simulink model "StartBlock"  (R2021b)
settings: Solver=VariableStepAuto  StartTime=0.0  StopTime=168  RelTol=1e-3  EnableMultiTasking=on
InitFcn:
  | % Load the model which describes
  | % the traffic flow throughout the
  | % day.
  | %load("TrafficFlowModel.Mat")
  | 
  | % Load the values at each quarter,
  | % Sufficient for traffic modelling.
  | load("TrafficFlowValues.mat")
undefined symbols (not defined in the file or in its folder): m, n, WhichPort
settings Model: Creator=Konrad  LastModifiedBy=Theodor Jonsson
settings SolverCC: AlgebraicLoopSolver=TrustRegion
settings DataIOCC: ReturnWorkspaceOutputs=off
settings OptimizationCC: LifeSpan=inf
settings DebuggingCC: SFUnexpectedBacktrackingDiag=warning  SFNoUnconditionalDefaultTransitionDiag=warning  SFExecutionAtInitializationDiag=none  SFMachineParentedDataDiag=warning  ArithmeticOperatorsInVariantConditions=warning
settings SFSimCC: SimUseLocalCustomCode=off  CustomCodeUndefinedFunction=UseInterfaceOnly
settings RTWCC: RTWUseLocalCustomCode=off
settings CodeAppCC: StateflowObjectComments=on
settings GRTTargetCC: TargetLangStandard=C89/C90 (ANSI)
settings ConfigComp: CovMetricSettings=dw  CovSaveCumulativeToWorkspaceVar=on  CovSaveSingleToWorkspaceVar=on  CovExternalEMLEnable=off

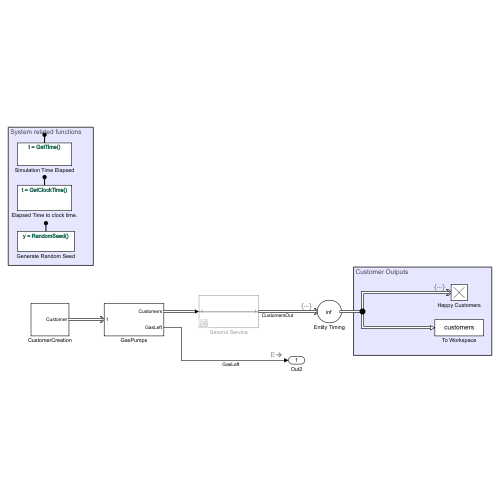
[thumbnail: Simulink's stored preview of the top-level diagram]
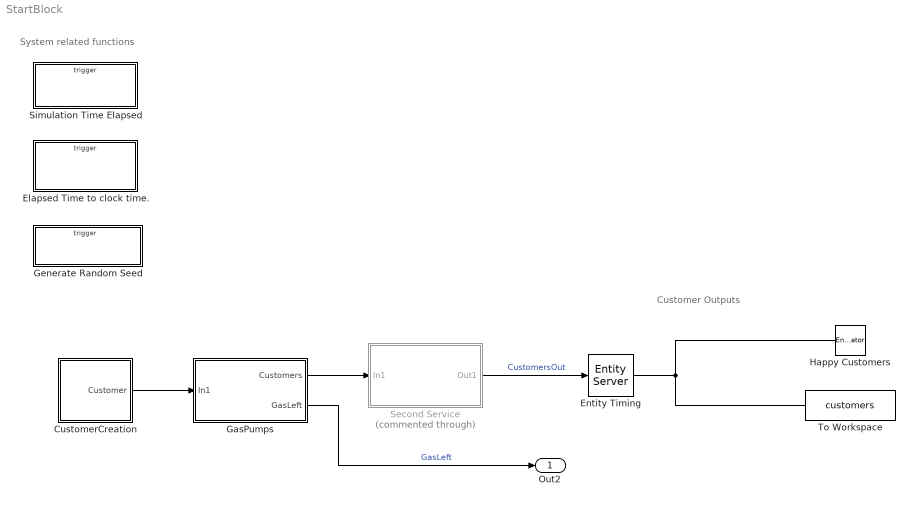
== system StartBlock ==
  note: Customer Outputs
  note: System related functions
  CustomerCreation : Subsystem  mask{mu_passengers=1.45, hunger_prob=0.4, mu_customers=150}
      mask prompts: mu_passengers "Average number of passengers"; hunger_prob "Probability one passenger hungry"; mu_customers "Arriving Customers per hour"
      mask DialogControl DescGroupVar Prompt: Entity Creation
  Elapsed Time to clock time. : Subsystem  TreatAsAtomicUnit=on
  Entity Timing : EntityServer  InputPortMessageModes=m  OutputPortMessageModes=m  Capacity=inf  ServiceTimeValue=0  EntryAction=entity.ServiceTime = GetTime()-entity.ServiceTime;
  GasPumps : Subsystem  mask{n_pumps=20, pump_rate=1200, tank_size=800000, que_cap=2}
      mask prompts: n_pumps "# Pumps"; pump_rate "Pump rate (l/h)"; tank_size "Tank Size"; que_cap "Per pump que capacity"
      mask DialogControl DescGroupVar Prompt: Gas Station
  Generate Random Seed : Subsystem  TreatAsAtomicUnit=on
  Happy Customers : EntityTerminator  InputPortMessageModes=m  EntryAction=entity.ServiceTime = GetTime()-entity.ServiceTime;
  Second Service : Subsystem  Commented=through
  Simulation Time Elapsed : Subsystem  TreatAsAtomicUnit=on
  To Workspace : ToWorkspace  VariableName=customers  SaveFormat=Timeseries  SampleTime=-1
  Out2 : Outport
  wires:
  GasPumps/1(Customers) -> Second Service/1(In1)
  Second Service/1(Out1) -> Entity Timing/1  "CustomersOut"
  GasPumps/2(GasLeft) -> Out2/1  "GasLeft"
  Entity Timing/1 -> Happy Customers/1, To Workspace/1
  CustomerCreation/1(Customer) -> GasPumps/1(In1)

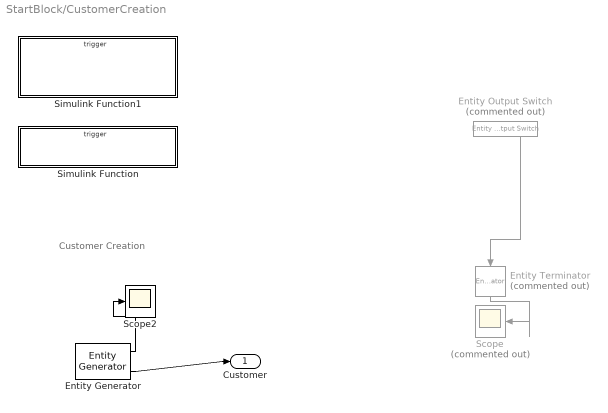
== system StartBlock/CustomerCreation ==
  note: Customer Creation
  Entity Output Switch : EntityOutputSwitch  Commented=on  InputPortMessageModes=m,m  OutputPortMessageModes=m,m  SwitchingCriterion=From control port  SwitchAttributeName=RequiredGas
      settings: InputPortMap=u0,u1
  Entity Generator : EntityGenerator  OutputPortMessageModes=n,m  TimeSource=MATLAB action  Period=1/4  IntergenerationTimeAction=|  GenerateAction=|  AttributeName=Vehicle|Passengers|RequiredGas|Hungry|ServiceTime  AttributeInitialValue=1|1|1|1|0  NumberEntitiesDeparted=on  EntityType=Structured  EntityTypeName=Customer
      IntergenerationTimeAction=|
      | seed = RandomSeed();
      | rng(seed);
      | dt = exprnd(1/(mu_customers*CustomerFrequency()+eps),1);
      GenerateAction=|
      | seed = RandomSeed();
      | rng(seed);
      | vehicle = GenerateVehicle(); % 1 for gas vehicle, 0 for non gas.
      | % In europe the average car occupies 1.5 passengers.
      | % Therefor sample from weighted descrete variable.
      | passengers = max(poissrnd(mu_passengers),1);
      | % Gas required.
      | if vehicle==1 % Car
      |     required_gas = normrnd(45,4);
      | elseif vehicle==2 % Trucks
      |     required_gas = normrnd(757,40);
      | else % Pedestrians don't need gas.
      |     required_gas = 0;
      | end
      | 
      | % Probability of buying snacks increases with the 
      | % amount of passengers and the time of day.
      | % Mid day low, Midnight high probability.
      | 
      | % Assuming that each person has a 25% chance of
      | % wanting buy snacks. Approve snacks attempt if 
      | % more than half of the passengers want to buy snacks.
      | 
      | hungry = binornd(passengers,hunger_prob)>=ceil(passengers/2);
      | % Described in words this checks if more or equal to half
      | % of the passengers are hungry given a probability p of hunger.
      | entity.Vehicle = vehicle;
      | entity.Passengers = passengers;
      | entity.RequiredGas = required_gas;
      | entity.Hungry = double(hungry);
      settings: OutputPortMap=o0,o3
  Entity Terminator : EntityTerminator  Commented=on  InputPortMessageModes=m  NumberEntitiesArrived=on
      settings: OutputPortMap=o0
  Scope : Scope  Commented=on
  Scope2 : Scope
  Simulink Function : Subsystem  TreatAsAtomicUnit=on
  Simulink Function1 : Subsystem  TreatAsAtomicUnit=on
  Customer : Outport
  wires:
  Entity Generator/1 -> Scope2/1
  Entity Generator/2 -> Customer/1
  Entity Output Switch/2 -> Entity Terminator/1
  Entity Terminator/1 -> Scope/1

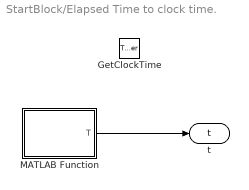
== system StartBlock/Elapsed Time to clock time. ==
  GetClockTime : TriggerPort  TriggerType=function-call  IsSimulinkFunction=on  FunctionName=GetClockTime  FunctionVisibility=scoped  VariantControl=(inherit)
  MATLAB Function : MATLAB Function  TreatAsAtomicUnit=on
  t : ArgOut  DisableCoverage=on  ArgumentName=t
  wires:
  MATLAB Function/1(T) -> t/1

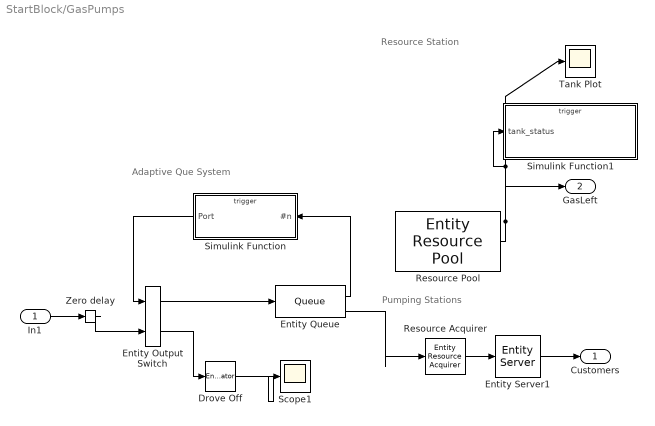
== system StartBlock/GasPumps ==
  note: Adaptive Que System
  note: Pumping Stations
  note: Resource Station
  In1 : Inport
  Drove Off : EntityTerminator  InputPortMessageModes=m  NumberEntitiesArrived=on
      settings: OutputPortMap=o0
  Entity Output Switch : EntityOutputSwitch  InputPortMessageModes=m,m  OutputPortMessageModes=m,m  SwitchingCriterion=From control port  SwitchAttributeName=Attribute1
      settings: InputPortMap=u0,u1
  Entity Queue : Queue  InputPortMessageModes=m  OutputPortMessageModes=n,m  Capacity=inf  EntryAction=entity.ServiceTime = GetTime();  NumberEntitiesInBlock=on
      settings: OutputPortMap=o1,o5
  Entity Server1 : EntityServer  InputPortMessageModes=m  OutputPortMessageModes=m  Capacity=n_pumps  ServiceTimeSource=MATLAB action  ServiceTimeValue=1  ServiceTimeAttributeName=RequiredGas  ServiceTimeAction=dt = entity.RequiredGas/pump_rate +0.1*(entity.RequiredGas>0);
  Resource Acquirer : EntityResourceAcquirer  InputPortMessageModes=m  OutputPortMessageModes=m  EntryAction=|  ResourceName=MainGasTank  ResourceAmountSource=Attribute  ResourceAmount=RequiredGas
      | gasleft = GasLeft();
      | if entity.RequiredGas > gasleft
      |     entity.RequiredGas = gasleft;    
      | end
      settings: OutputPortMap=o3
  Resource Pool : EntityResourcePool  ResourceName=MainGasTank  ReusableUponRelease=off  ResourceGranularity=Fractional amount  ResourceAmount=tank_size  AmountAvailable=on
      settings: OutputPortMap=o2
  Scope1 : Scope
  Simulink Function : Subsystem  TreatAsAtomicUnit=on
  Simulink Function1 : Subsystem  TreatAsAtomicUnit=on
  Tank Plot : Scope
  Zero delay : EntityServer  InputPortMessageModes=m  OutputPortMessageModes=m  Capacity=inf  ServiceTimeValue=0  EntryAction=WhichPort()
  Customers : Outport  VectorParamsAs1DForOutWhenUnconnected=off
  GasLeft : Outport  Port=2
  wires:
  In1/1 -> Zero delay/1
  Entity Queue/1 -> Simulink Function/1(#n)
  Simulink Function/1(Port) -> Entity Output Switch/1
  Entity Queue/2 -> Resource Acquirer/1
  Entity Output Switch/1 -> Entity Queue/1
  Entity Output Switch/2 -> Drove Off/1
  Zero delay/1 -> Entity Output Switch/2
  Entity Server1/1 -> Customers/1
  Resource Acquirer/1 -> Entity Server1/1
  Resource Pool/1 -> Tank Plot/1, Simulink Function1/1(tank_status), GasLeft/1
  Drove Off/1 -> Scope1/1

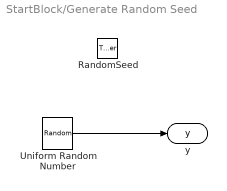
== system StartBlock/Generate Random Seed ==
  RandomSeed : TriggerPort  TriggerType=function-call  IsSimulinkFunction=on  FunctionName=RandomSeed  FunctionVisibility=scoped  VariantControl=(inherit)
  Uniform Random Number : UniformRandomNumber  Minimum=100000  Maximum=1000000000  Seed=randi(10000000)
  y : ArgOut  DisableCoverage=on  ArgumentName=y
  wires:
  Uniform Random Number/1 -> y/1

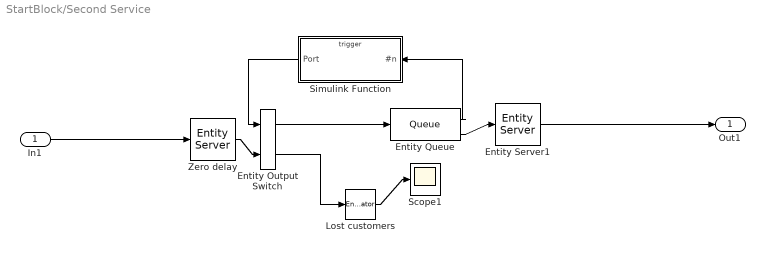
== system StartBlock/Second Service ==
  In1 : Inport
  Entity Output Switch : EntityOutputSwitch  InputPortMessageModes=m,m  OutputPortMessageModes=m,m  SwitchingCriterion=From control port  SwitchAttributeName=Attribute1
      settings: InputPortMap=u0,u1
  Entity Queue : Queue  InputPortMessageModes=m  OutputPortMessageModes=n,m  NumberEntitiesInBlock=on
      settings: OutputPortMap=o1,o5
  Entity Server1 : EntityServer  InputPortMessageModes=m  OutputPortMessageModes=m  Capacity=1
  Lost customers : EntityTerminator  InputPortMessageModes=m  NumberEntitiesArrived=on
      settings: OutputPortMap=o0
  Scope1 : Scope
  Simulink Function : Subsystem  TreatAsAtomicUnit=on
  Zero delay : EntityServer  InputPortMessageModes=m  OutputPortMessageModes=m  Capacity=inf  ServiceTimeValue=0  EntryAction=WhichPort()
  Out1 : Outport  VectorParamsAs1DForOutWhenUnconnected=off
  wires:
  In1/1 -> Zero delay/1
  Entity Queue/1 -> Simulink Function/1(#n)
  Simulink Function/1(Port) -> Entity Output Switch/1
  Entity Queue/2 -> Entity Server1/1
  Entity Server1/1 -> Out1/1
  Lost customers/1 -> Scope1/1
  Entity Output Switch/1 -> Entity Queue/1
  Entity Output Switch/2 -> Lost customers/1
  Zero delay/1 -> Entity Output Switch/2

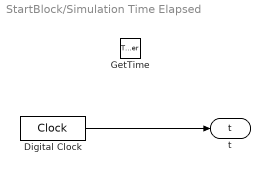
== system StartBlock/Simulation Time Elapsed ==
  GetTime : TriggerPort  TriggerType=function-call  IsSimulinkFunction=on  FunctionName=GetTime  FunctionVisibility=scoped  VariantControl=(inherit)
  Digital Clock : DigitalClock  SampleTime=-1
  t : ArgOut  DisableCoverage=on  ArgumentName=t
  wires:
  Digital Clock/1 -> t/1

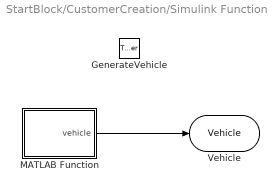
== system StartBlock/CustomerCreation/Simulink Function ==
  GenerateVehicle : TriggerPort  TriggerType=function-call  IsSimulinkFunction=on  FunctionName=GenerateVehicle  FunctionVisibility=scoped  VariantControl=(inherit)
  MATLAB Function : MATLAB Function  TreatAsAtomicUnit=on
  Vehicle : ArgOut  DisableCoverage=on  ArgumentName=Vehicle
  wires:
  MATLAB Function/1(vehicle) -> Vehicle/1

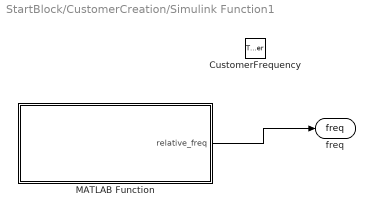
== system StartBlock/CustomerCreation/Simulink Function1 ==
  CustomerFrequency : TriggerPort  TriggerType=function-call  IsSimulinkFunction=on  FunctionName=CustomerFrequency  FunctionVisibility=scoped  VariantControl=(inherit)
  MATLAB Function : MATLAB Function  TreatAsAtomicUnit=on
  freq : ArgOut  DisableCoverage=on  ArgumentName=freq
  wires:
  MATLAB Function/1(relative_freq) -> freq/1

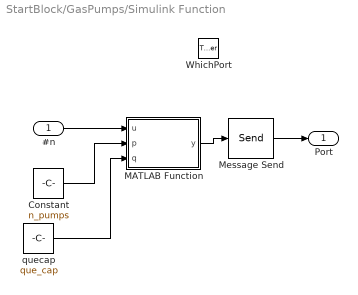
== system StartBlock/GasPumps/Simulink Function ==
  #n : Inport
  WhichPort : TriggerPort  TriggerType=function-call  IsSimulinkFunction=on  FunctionName=WhichPort  FunctionVisibility=scoped  VariantControl=Variant
  Constant : Constant  Value=n_pumps  SampleTime=-1
  MATLAB Function : MATLAB Function  TreatAsAtomicUnit=on
  Message Send : Send  OutputPortMessageModes=m
  quecap : Constant  Value=que_cap  SampleTime=-1
  Port : Outport  VectorParamsAs1DForOutWhenUnconnected=off
  wires:
  Message Send/1 -> Port/1
  #n/1 -> MATLAB Function/1(u)
  MATLAB Function/1(y) -> Message Send/1
  Constant/1 -> MATLAB Function/2(p)
  quecap/1 -> MATLAB Function/3(q)

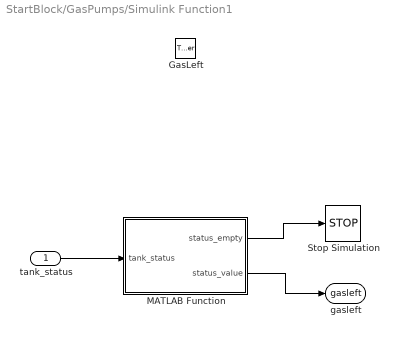
== system StartBlock/GasPumps/Simulink Function1 ==
  tank_status : Inport
  GasLeft : TriggerPort  TriggerType=function-call  IsSimulinkFunction=on  FunctionName=GasLeft  FunctionVisibility=scoped  VariantControl=(inherit)
  MATLAB Function : MATLAB Function  TreatAsAtomicUnit=on
  Stop Simulation : Stop
  gasleft : ArgOut  DisableCoverage=on  ArgumentName=gasleft
  wires:
  MATLAB Function/1(status_empty) -> Stop Simulation/1
  MATLAB Function/2(status_value) -> gasleft/1
  tank_status/1 -> MATLAB Function/1(tank_status)

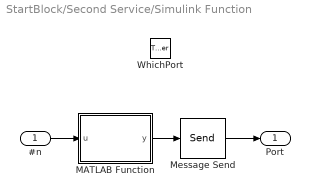
== system StartBlock/Second Service/Simulink Function ==
  #n : Inport
  WhichPort : TriggerPort  TriggerType=function-call  IsSimulinkFunction=on  FunctionName=WhichPort  FunctionVisibility=scoped  VariantControl=Variant
  MATLAB Function : MATLAB Function  TreatAsAtomicUnit=on
  Message Send : Send  OutputPortMessageModes=m
  Port : Outport  VectorParamsAs1DForOutWhenUnconnected=off
  wires:
  Message Send/1 -> Port/1
  #n/1 -> MATLAB Function/1(u)
  MATLAB Function/1(y) -> Message Send/1

== matlab function StartBlock/GasPumps/Simulink Function/MATLAB Function ==
  data: u input; y output; p input; q input
function y = fcn(u,p,q)

limit=q*p;
if u<limit
    y=1;
else
    y=2;
end

== matlab function StartBlock/GasPumps/Simulink Function1/MATLAB Function ==
  data: status_empty output; status_value output; tank_status input
function [status_empty,status_value] = fcn(tank_status)
% Check if the resourse tank is empty.
% The system will terminate if the tank is empty.
% 
% INPUT:
%   
%   tank_status - The number of liters left in the tank.
%
% OUTPUT:
%   
%   status_empty - 1 if empty 0 else.
%
%   status_value - Number of liters left.
%

status_empty = tank_status<=0;
status_value = tank_status;
end

== matlab function StartBlock/CustomerCreation/Simulink Function/MATLAB Function ==
  data: vehicle output
function vehicle = GenVehicle()
% GENVEHICLE Generates a vehicle representation at depending on time of
%   day. 1 for PassengerCar, 2 for semi.
%
% INPUT
%   ...
%
% OUTPUT
%
%   vehicle - (int) Representation of time.
%
T = GetClockTime();
% The frequency of the vehicle depends on time.
% The following have been used:
%   CARS in TRUCK
%    50       1   04.00->21.00
%    30       1   21.00->02.00
%    10       1   02.00->04.00
if T>=4 && T<21
    p_semi = 1/50;
elseif T>=21 || T<2
    p_semi = 1/30;
else
    p_semi = 1/10;
end

% We now sample the vehicle type using randsample
vehicle = randsample([1,2],1,true,[1-p_semi,p_semi]);
end

== matlab function StartBlock/Elapsed Time to clock time./MATLAB Function ==
  data: T output
function T = ElapsedToClock()
% TIMETOCLOCK Converts the elapsed time of the simulation to clock time.
%
% INPUT
%   ...
% OUTPUT
%   
%   T - Time of the day, i.e. 4 PM or 16.00
%
T = GetTime();
T = mod(T,24);
end

== matlab function StartBlock/CustomerCreation/Simulink Function1/MATLAB Function ==
  data: relative_freq output; traffic_values parameter
function relative_freq = InspectFrequency(traffic_values)
    % traffic_values is taken from matlab workspace and loaded
    % during InitFcn for the model.
    T = GetClockTime();
    t = round(T*4)/4;
    relative_freq = traffic_values(t*4+1);
end

== matlab function StartBlock/Second Service/Simulink Function/MATLAB Function ==
  data: u input; y output
function y = fcn(u)
%#codegen
LimitValue=2;
if u<LimitValue
    y=1;
else
    y=2;
end
